simulink model "DYN_01x"  (R2018b)
settings: Solver=FixedStepAuto  StartTime=0.0  StopTime=100  FixedStep=0.01  RelTol=1e-3
(part 1 of 13)
settings Model: Creator=TMP  LastModifiedBy=TMP
settings DataIOCC: ReturnWorkspaceOutputs=on

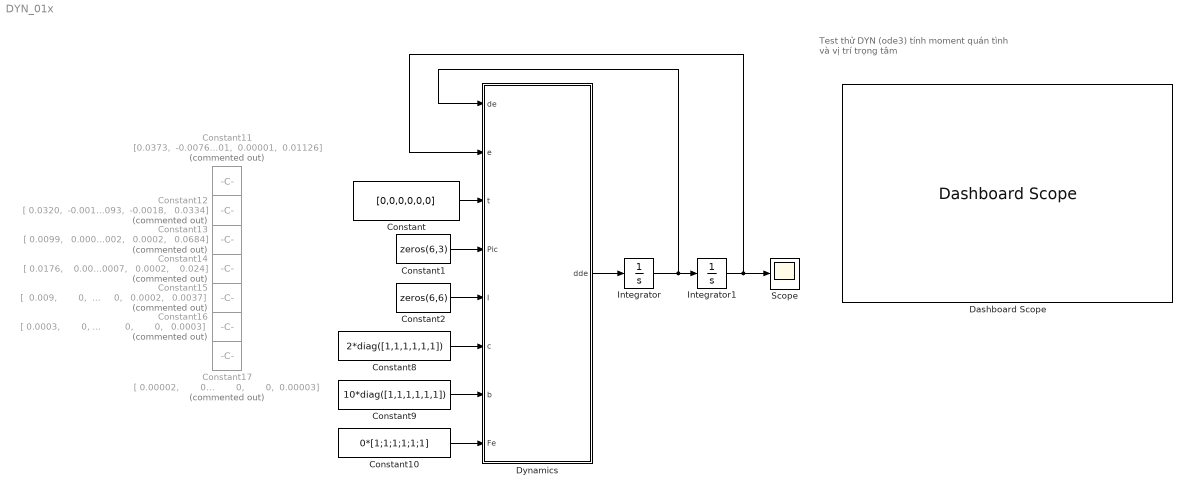
== system DYN_01x ==
  note: Test thử DYN (ode3)
      | tính moment quán tình và vị trí trọng tâm
  Constant : Constant  Value=[0,0,0,0,0,0]
  Constant1 : Constant  Value=zeros(6,3)
  Constant10 : Constant  Value=0*[1;1;1;1;1;1]
  Constant11 : Constant  Commented=on  Value=|
      | [0.0373,  -0.0076,   0.1064;
      |        0.1127,   0.0065,   0.0648;
      |        0.0447,   0.0125,  -0.0554;
      |        0.0006,   0.0052,   0.1068;
      |             0,   0.0062,   0.0195;
      |      -0.00001,  0.00001,  0.01126]
  Constant12 : Constant  Commented=on  Value=|
      | [ 0.0320,  -0.0017,   0.0093;
      |       -0.0017,   0.0364,  -0.0018;
      |        0.0093,  -0.0018,   0.0334]
  Constant13 : Constant  Commented=on  Value=|
      | [ 0.0099,   0.0008,  -0.0002;
      |        0.0008,   0.0646,   0.0002;
      |       -0.0002,   0.0002,   0.0684]
  Constant14 : Constant  Commented=on  Value=|
      | [ 0.0176,    0.001,   0.0007;
      |         0.001,   0.0195,   0.0002;
      |        0.0007,   0.0002,    0.024]
  Constant15 : Constant  Commented=on  Value=|
      | [  0.009,        0,        0;
      |             0,   0.0081,   0.0002;
      |             0,   0.0002,   0.0037]
  Constant16 : Constant  Commented=on  Value=|
      | [ 0.0003,        0,        0;
      |             0,   0.0002,        0;
      |             0,        0,   0.0003]
  Constant17 : Constant  Commented=on  Value=|
      | [ 0.00002,        0,        0;
      |              0,  0.00002,        0;
      |              0,        0,  0.00003]
  Constant2 : Constant  Value=zeros(6,6)
  Constant8 : Constant  Value=2*diag([1,1,1,1,1,1])
  Constant9 : Constant  Value=10*diag([1,1,1,1,1,1])
  Dashboard Scope : DashboardScope  WebBlockId=9
  Dynamics : MATLAB Function  TreatAsAtomicUnit=on
  Integrator : Integrator  InitialCondition=[0;0;0;0;0;0]
  Integrator1 : Integrator  InitialCondition=[0;0;0;0;0;0]
  Scope : Scope
  wires:
  Dynamics/1(dde) -> Integrator/1
  Integrator/1 -> Dynamics/1(de), Integrator1/1
  Integrator1/1 -> Dynamics/2(e), Scope/1
  Constant1/1 -> Dynamics/4(Pic)
  Constant8/1 -> Dynamics/6(c)
  Constant9/1 -> Dynamics/7(b)
  Constant10/1 -> Dynamics/8(Fe)
  Constant2/1 -> Dynamics/5(I)
  Constant/1 -> Dynamics/3(t)
